simulink model "SF005A_StOutpCtrl"  (R2013b)
settings: Solver=FixedStepDiscrete  SolverMode=SingleTasking  StartTime=0.0  StopTime=1  FixedStep=0.002  RelTol=1e-3
values from neighbouring files (symbols this model uses):
  ARCHGLBPRM_2MILLISEC_SEC_F32 = DataDict.Constant    [SF005A_StOutpCtrl_DataDict.m]
  ARCHGLBPRM_FLOATZEROTHD_ULS_F32 = DataDict.Constant    [SF005A_StOutpCtrl_DataDict.m]
  BIGSLEW_ULSPERSEC_F32 = DataDict.Constant    [SF005A_StOutpCtrl_DataDict.m]
  DI_CNT_U08 = DataDict.Constant    [SF005A_StOutpCtrl_DataDict.m]
  LOA_CNT_U08 = DataDict.Constant    [SF005A_StOutpCtrl_DataDict.m]
  OPER_CNT_U08 = DataDict.Constant    [SF005A_StOutpCtrl_DataDict.m]
  STRTSTOP_CNT_U08 = DataDict.Constant    [SF005A_StOutpCtrl_DataDict.m]
libraries: NxtrLim x3, simulink x2, NxtrAbslt x1
(part 2 of 2)

== system SF005A_StOutpCtrl/StOutpCtrl/StOutpCtrlPer1/Target Selection/RateLimit ==
  note: v1.4.0: Replaced case 3 with default.
  RateSource : Inport
  OperRateLimit : Inport  Port=2
  LoaRateLimit : Inport  Port=3
  StrtStopRateLimit : Inport  Port=4
  CopyRight2 : Subsystem  Description=|  mask(Copyright Information){none=on}
      | Copyright info block.                                               
      |                                                                     
      | Place copyright information at the top of every subsystem in design.
      mask prompts: none "No parameters"
      mask help: Place copyright information at the top of every subsystem in design.
      mask Display:
      | NxtrConf = 'Nexteer Confidential';
      | 
      | sys = bdroot; %handle for the current model ("system")
      | first = get_param(sys,'Created');
      | first = first(end-3:end);  %year is last four digits
      | 
      | last = get_param(sys,'LastModifiedDate');
      | if isempty(last)
      |     last = datestr(now,'yyyy');
      | else
      |     last = last(end-3:end);
      | end
      | 
      | if strcmp(first,last)
      |     fprintf('%s -- Copyright %s Nexteer',NxtrConf,first)
      | else
      |     fprintf('%s -- %s%s- %s Nexteer',NxtrConf,char(169),first,last)
      | end
  Loa : Subsystem  TreatAsAtomicUnit=on
  Merge : Merge  Inputs=3
  Oper : Subsystem  TreatAsAtomicUnit=on
  StrtStop : Subsystem  TreatAsAtomicUnit=on
  Switch Case : SwitchCase  CaseConditions={1,2}
      settings: AttributesFormatString=|
      | Case 1: Oper
      | Case 2: Loa
      | Case 3: StrtStop
  RateLim : Outport
  wires:
  RateSource/1 -> Switch Case/1
  OperRateLimit/1 -> Oper/1(In1)
  StrtStopRateLimit/1 -> StrtStop/1(In1)
  Merge/1 -> RateLim/1  "SelectedRampRate_UlsPerSec_T_f32"
  StrtStop/1(Out1) -> Merge/1
  Loa/1(Out1) -> Merge/2
  LoaRateLimit/1 -> Loa/1(In1)
  Switch Case/1 -> Oper/Action
  Switch Case/2 -> Loa/Action
  Switch Case/3 -> StrtStop/Action
  Oper/1(Out1) -> Merge/3

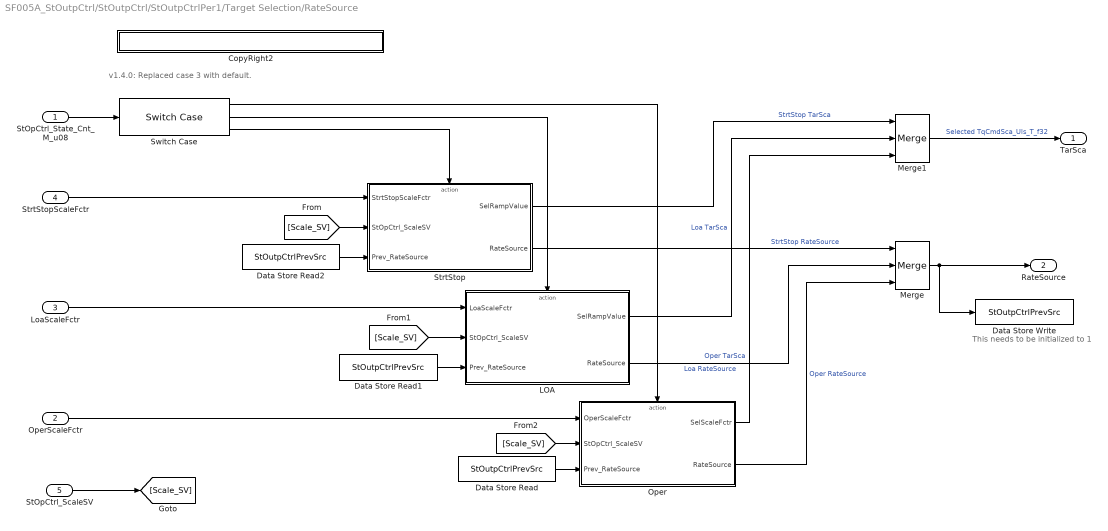
== system SF005A_StOutpCtrl/StOutpCtrl/StOutpCtrlPer1/Target Selection/RateSource ==
  note: v1.4.0: Replaced case 3 with default.
  note: This needs to be initialized to 1
  StOpCtrl_State_Cnt_M_u08 : Inport
  OperScaleFctr : Inport  Port=2
  LoaScaleFctr : Inport  Port=3
  StrtStopScaleFctr : Inport  Port=4
  StOpCtrl_ScaleSV : Inport  Port=5
  CopyRight2 : Subsystem  Description=|  mask(Copyright Information){none=on}
      | Copyright info block.                                               
      |                                                                     
      | Place copyright information at the top of every subsystem in design.
      mask prompts: none "No parameters"
      mask help: Place copyright information at the top of every subsystem in design.
      mask Display:
      | NxtrConf = 'Nexteer Confidential';
      | 
      | sys = bdroot; %handle for the current model ("system")
      | first = get_param(sys,'Created');
      | first = first(end-3:end);  %year is last four digits
      | 
      | last = get_param(sys,'LastModifiedDate');
      | if isempty(last)
      |     last = datestr(now,'yyyy');
      | else
      |     last = last(end-3:end);
      | end
      | 
      | if strcmp(first,last)
      |     fprintf('%s -- Copyright %s Nexteer',NxtrConf,first)
      | else
      |     fprintf('%s -- %s%s- %s Nexteer',NxtrConf,char(169),first,last)
      | end
  Data Store Read : DataStoreRead  DataStoreName=StOutpCtrlPrevSrc
  Data Store Read1 : DataStoreRead  DataStoreName=StOutpCtrlPrevSrc
  Data Store Read2 : DataStoreRead  DataStoreName=StOutpCtrlPrevSrc
  Data Store Write : DataStoreWrite  DataStoreName=StOutpCtrlPrevSrc
  LOA : Subsystem
  Merge : Merge  Inputs=3
  Merge1 : Merge  Inputs=3
  Oper : Subsystem
  StrtStop : Subsystem
  Switch Case : SwitchCase  CaseConditions={1,2}
      settings: AttributesFormatString=|
      | case 1: Oper
      | case 2: Loa
      | case 3: StrtStop
  TarSca : Outport
  RateSource : Outport  Port=2
  wires:
  Merge1/1 -> TarSca/1  "Selected TqCmdSca_Uls_T_f32"
  Oper/1(SelScaleFctr) -> Merge1/3  "Oper TarSca"
  LOA/2(RateSource) -> Merge/2  "Loa RateSource"
  LOA/1(SelRampValue) -> Merge1/2  "Loa TarSca"
  StrtStop/1(SelRampValue) -> Merge1/1  "StrtStop TarSca"
  Switch Case/1 -> Oper/Action
  Switch Case/2 -> LOA/Action
  Switch Case/3 -> StrtStop/Action
  Data Store Read2/1 -> StrtStop/3(Prev_RateSource)
  Data Store Read1/1 -> LOA/3(Prev_RateSource)
  [Scale_SV] -> Oper/2(StOpCtrl_ScaleSV)
  [Scale_SV] -> LOA/2(StOpCtrl_ScaleSV)
  [Scale_SV] -> StrtStop/2(StOpCtrl_ScaleSV)
  StOpCtrl_ScaleSV/1 -> [Scale_SV]
  StOpCtrl_State_Cnt_M_u08/1 -> Switch Case/1
  Oper/2(RateSource) -> Merge/3  "Oper RateSource"
  StrtStop/2(RateSource) -> Merge/1  "StrtStop RateSource"
  Merge/1 -> Data Store Write/1, RateSource/1
  StrtStopScaleFctr/1 -> StrtStop/1(StrtStopScaleFctr)
  OperScaleFctr/1 -> Oper/1(OperScaleFctr)
  LoaScaleFctr/1 -> LOA/1(LoaScaleFctr)
  Data Store Read/1 -> Oper/3(Prev_RateSource)

== system SF005A_StOutpCtrl/StOutpCtrl/StOutpCtrlPer1/Diag Override/If Action Subsystem6/CopyRight2 ==

== system SF005A_StOutpCtrl/StOutpCtrl/StOutpCtrlPer1/Diag Override/If Action Subsystem7/CopyRight2 ==

== system SF005A_StOutpCtrl/StOutpCtrl/StOutpCtrlPer1/System State Request /CtrldShtDwnFlt_FALSE/CopyRight2 ==

== system SF005A_StOutpCtrl/StOutpCtrl/StOutpCtrlPer1/System State Request /CtrldShtDwnFlt_TRUE/CopyRight2 ==

== system SF005A_StOutpCtrl/StOutpCtrl/StOutpCtrlPer1/System State Request /RampCmpl_FALSE/CopyRight2 ==

== system SF005A_StOutpCtrl/StOutpCtrl/StOutpCtrlPer1/System State Request /RampCmpl_TRUE/CopyRight2 ==

== system SF005A_StOutpCtrl/StOutpCtrl/StOutpCtrlPer1/Target Selection/RampValue/CopyRight2 ==

== system SF005A_StOutpCtrl/StOutpCtrl/StOutpCtrlPer1/Target Selection/RampValue/LOA ==
  Action Port : ActionPort  ActionType=elseif
  Constant1 : Constant  Value=LOA_CNT_U08  OutDataTypeStr=uint8
      settings: AttributesFormatString=%<OutDataTypeStr>
  CopyRight2 : Subsystem  Description=|  mask(Copyright Information){none=on}
      | Copyright info block.                                               
      |                                                                     
      | Place copyright information at the top of every subsystem in design.
      mask prompts: none "No parameters"
      mask help: Place copyright information at the top of every subsystem in design.
      mask Display:
      | NxtrConf = 'Nexteer Confidential';
      | 
      | sys = bdroot; %handle for the current model ("system")
      | first = get_param(sys,'Created');
      | first = first(end-3:end);  %year is last four digits
      | 
      | last = get_param(sys,'LastModifiedDate');
      | if isempty(last)
      |     last = datestr(now,'yyyy');
      | else
      |     last = last(end-3:end);
      | end
      | 
      | if strcmp(first,last)
      |     fprintf('%s -- Copyright %s Nexteer',NxtrConf,first)
      | else
      |     fprintf('%s -- %s%s- %s Nexteer',NxtrConf,char(169),first,last)
      | end
  Out1 : Outport
  wires:
  Constant1/1 -> Out1/1

== system SF005A_StOutpCtrl/StOutpCtrl/StOutpCtrlPer1/Target Selection/RampValue/Oper ==
  Action Port : ActionPort  ActionType=else
  Constant : Constant  Value=OPER_CNT_U08  OutDataTypeStr=uint8
      settings: AttributesFormatString=%<OutDataTypeStr>
  CopyRight2 : Subsystem  Description=|  mask(Copyright Information){none=on}
      | Copyright info block.                                               
      |                                                                     
      | Place copyright information at the top of every subsystem in design.
      mask prompts: none "No parameters"
      mask help: Place copyright information at the top of every subsystem in design.
      mask Display:
      | NxtrConf = 'Nexteer Confidential';
      | 
      | sys = bdroot; %handle for the current model ("system")
      | first = get_param(sys,'Created');
      | first = first(end-3:end);  %year is last four digits
      | 
      | last = get_param(sys,'LastModifiedDate');
      | if isempty(last)
      |     last = datestr(now,'yyyy');
      | else
      |     last = last(end-3:end);
      | end
      | 
      | if strcmp(first,last)
      |     fprintf('%s -- Copyright %s Nexteer',NxtrConf,first)
      | else
      |     fprintf('%s -- %s%s- %s Nexteer',NxtrConf,char(169),first,last)
      | end
  Out1 : Outport
  wires:
  Constant/1 -> Out1/1

== system SF005A_StOutpCtrl/StOutpCtrl/StOutpCtrlPer1/Target Selection/RampValue/StrtStop ==
  Action Port : ActionPort  ActionType=then
  Constant2 : Constant  Value=STRTSTOP_CNT_U08  OutDataTypeStr=uint8
      settings: AttributesFormatString=%<OutDataTypeStr>
  CopyRight2 : Subsystem  Description=|  mask(Copyright Information){none=on}
      | Copyright info block.                                               
      |                                                                     
      | Place copyright information at the top of every subsystem in design.
      mask prompts: none "No parameters"
      mask help: Place copyright information at the top of every subsystem in design.
      mask Display:
      | NxtrConf = 'Nexteer Confidential';
      | 
      | sys = bdroot; %handle for the current model ("system")
      | first = get_param(sys,'Created');
      | first = first(end-3:end);  %year is last four digits
      | 
      | last = get_param(sys,'LastModifiedDate');
      | if isempty(last)
      |     last = datestr(now,'yyyy');
      | else
      |     last = last(end-3:end);
      | end
      | 
      | if strcmp(first,last)
      |     fprintf('%s -- Copyright %s Nexteer',NxtrConf,first)
      | else
      |     fprintf('%s -- %s%s- %s Nexteer',NxtrConf,char(169),first,last)
      | end
  Out1 : Outport
  wires:
  Constant2/1 -> Out1/1

== system SF005A_StOutpCtrl/StOutpCtrl/StOutpCtrlPer1/Target Selection/RateLimit/CopyRight2 ==

== system SF005A_StOutpCtrl/StOutpCtrl/StOutpCtrlPer1/Target Selection/RateLimit/Loa ==
  In1 : Inport
  Action Port : ActionPort  ActionType=case
  CopyRight2 : Subsystem  Description=|  mask(Copyright Information){none=on}
      | Copyright info block.                                               
      |                                                                     
      | Place copyright information at the top of every subsystem in design.
      mask prompts: none "No parameters"
      mask help: Place copyright information at the top of every subsystem in design.
      mask Display:
      | NxtrConf = 'Nexteer Confidential';
      | 
      | sys = bdroot; %handle for the current model ("system")
      | first = get_param(sys,'Created');
      | first = first(end-3:end);  %year is last four digits
      | 
      | last = get_param(sys,'LastModifiedDate');
      | if isempty(last)
      |     last = datestr(now,'yyyy');
      | else
      |     last = last(end-3:end);
      | end
      | 
      | if strcmp(first,last)
      |     fprintf('%s -- Copyright %s Nexteer',NxtrConf,first)
      | else
      |     fprintf('%s -- %s%s- %s Nexteer',NxtrConf,char(169),first,last)
      | end
  Out1 : Outport
  wires:
  In1/1 -> Out1/1

== system SF005A_StOutpCtrl/StOutpCtrl/StOutpCtrlPer1/Target Selection/RateLimit/Oper ==
  In1 : Inport
  Action Port : ActionPort  ActionType=case
  CopyRight2 : Subsystem  Description=|  mask(Copyright Information){none=on}
      | Copyright info block.                                               
      |                                                                     
      | Place copyright information at the top of every subsystem in design.
      mask prompts: none "No parameters"
      mask help: Place copyright information at the top of every subsystem in design.
      mask Display:
      | NxtrConf = 'Nexteer Confidential';
      | 
      | sys = bdroot; %handle for the current model ("system")
      | first = get_param(sys,'Created');
      | first = first(end-3:end);  %year is last four digits
      | 
      | last = get_param(sys,'LastModifiedDate');
      | if isempty(last)
      |     last = datestr(now,'yyyy');
      | else
      |     last = last(end-3:end);
      | end
      | 
      | if strcmp(first,last)
      |     fprintf('%s -- Copyright %s Nexteer',NxtrConf,first)
      | else
      |     fprintf('%s -- %s%s- %s Nexteer',NxtrConf,char(169),first,last)
      | end
  Out1 : Outport
  wires:
  In1/1 -> Out1/1

== system SF005A_StOutpCtrl/StOutpCtrl/StOutpCtrlPer1/Target Selection/RateLimit/StrtStop ==
  In1 : Inport
  Action Port : ActionPort  ActionType=case
  CopyRight2 : Subsystem  Description=|  mask(Copyright Information){none=on}
      | Copyright info block.                                               
      |                                                                     
      | Place copyright information at the top of every subsystem in design.
      mask prompts: none "No parameters"
      mask help: Place copyright information at the top of every subsystem in design.
      mask Display:
      | NxtrConf = 'Nexteer Confidential';
      | 
      | sys = bdroot; %handle for the current model ("system")
      | first = get_param(sys,'Created');
      | first = first(end-3:end);  %year is last four digits
      | 
      | last = get_param(sys,'LastModifiedDate');
      | if isempty(last)
      |     last = datestr(now,'yyyy');
      | else
      |     last = last(end-3:end);
      | end
      | 
      | if strcmp(first,last)
      |     fprintf('%s -- Copyright %s Nexteer',NxtrConf,first)
      | else
      |     fprintf('%s -- %s%s- %s Nexteer',NxtrConf,char(169),first,last)
      | end
  Out1 : Outport
  wires:
  In1/1 -> Out1/1

== system SF005A_StOutpCtrl/StOutpCtrl/StOutpCtrlPer1/Target Selection/RateSource/CopyRight2 ==

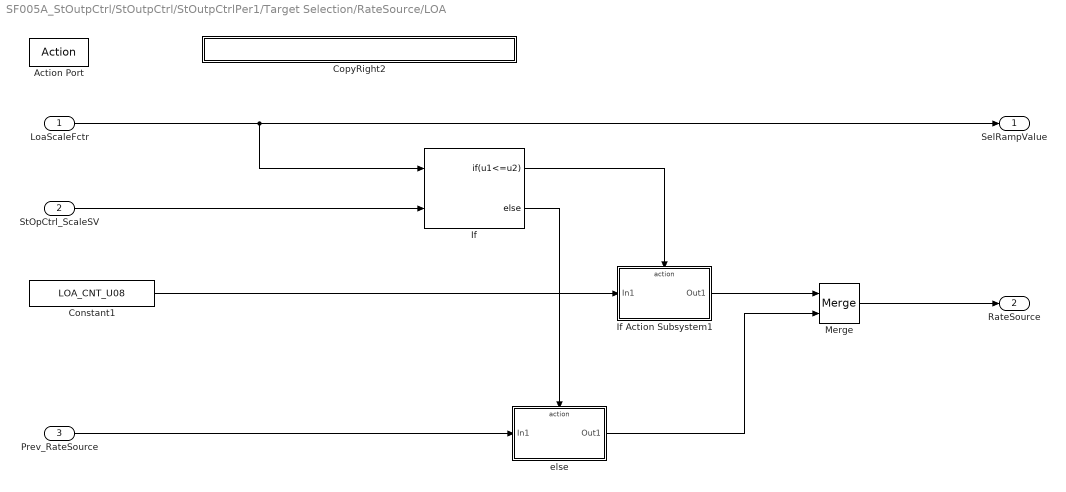
== system SF005A_StOutpCtrl/StOutpCtrl/StOutpCtrlPer1/Target Selection/RateSource/LOA ==
  LoaScaleFctr : Inport
  StOpCtrl_ScaleSV : Inport  Port=2
  Prev_RateSource : Inport  Port=3
  Action Port : ActionPort  ActionType=case
  Constant1 : Constant  Value=LOA_CNT_U08  OutDataTypeStr=uint8
      settings: AttributesFormatString=%<OutDataTypeStr>
  CopyRight2 : Subsystem  Description=|  mask(Copyright Information){none=on}
      | Copyright info block.                                               
      |                                                                     
      | Place copyright information at the top of every subsystem in design.
      mask prompts: none "No parameters"
      mask help: Place copyright information at the top of every subsystem in design.
      mask Display:
      | NxtrConf = 'Nexteer Confidential';
      | 
      | sys = bdroot; %handle for the current model ("system")
      | first = get_param(sys,'Created');
      | first = first(end-3:end);  %year is last four digits
      | 
      | last = get_param(sys,'LastModifiedDate');
      | if isempty(last)
      |     last = datestr(now,'yyyy');
      | else
      |     last = last(end-3:end);
      | end
      | 
      | if strcmp(first,last)
      |     fprintf('%s -- Copyright %s Nexteer',NxtrConf,first)
      | else
      |     fprintf('%s -- %s%s- %s Nexteer',NxtrConf,char(169),first,last)
      | end
  If : If  RequirementInfo={'linktype_rmi_doors' '0000baae (/E-STEER Core/SubSystem Specifications/Application Functions/SF005A State Output Control)' '#SF005A_54' 'true' 'REQ: SF005A_54' '' ; 'linktype_rmi_doors' '0000baae (/E-STEER Core/SubSystem Specifications/Application Functions/SF005A State Output Control)' '#SF005A_55' 'true' 'REQ: SF005A_55' '' ; 'linktype_rmi_doors' '0000baae (/E-STEER Core/SubSystem Specifications/Application Functions/SF005A State Output Control)' '#SF005A_61' 'true' 'REQ: SF005A_61' '' } %GIDa_5c692240_752d_457b_a676_1ce9a35b4c5b  NumInputs=2  IfExpression=u1<=u2
  If Action Subsystem1 : Subsystem  TreatAsAtomicUnit=on
  Merge : Merge
  else : Subsystem  TreatAsAtomicUnit=on
  SelRampValue : Outport
  RateSource : Outport  Port=2
  wires:
  If Action Subsystem1/1(Out1) -> Merge/1
  else/1(Out1) -> Merge/2
  Merge/1 -> RateSource/1
  Prev_RateSource/1 -> else/1(In1)
  If/2 -> else/Action
  Constant1/1 -> If Action Subsystem1/1(In1)
  StOpCtrl_ScaleSV/1 -> If/2
  If/1 -> If Action Subsystem1/Action
  LoaScaleFctr/1 -> If/1, SelRampValue/1

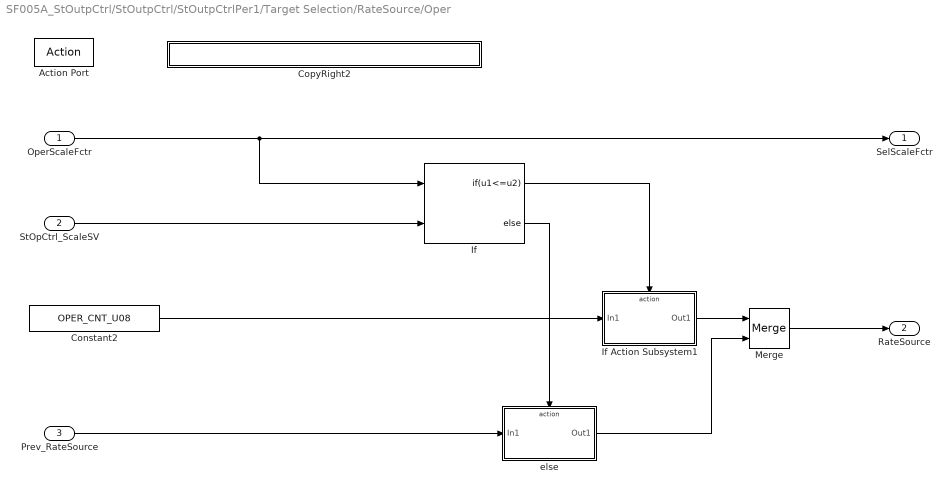
== system SF005A_StOutpCtrl/StOutpCtrl/StOutpCtrlPer1/Target Selection/RateSource/Oper ==
  OperScaleFctr : Inport
  StOpCtrl_ScaleSV : Inport  Port=2
  Prev_RateSource : Inport  Port=3
  Action Port : ActionPort  ActionType=case
  Constant2 : Constant  Value=OPER_CNT_U08  OutDataTypeStr=uint8
      settings: AttributesFormatString=%<OutDataTypeStr>
  CopyRight2 : Subsystem  Description=|  mask(Copyright Information){none=on}
      | Copyright info block.                                               
      |                                                                     
      | Place copyright information at the top of every subsystem in design.
      mask prompts: none "No parameters"
      mask help: Place copyright information at the top of every subsystem in design.
      mask Display:
      | NxtrConf = 'Nexteer Confidential';
      | 
      | sys = bdroot; %handle for the current model ("system")
      | first = get_param(sys,'Created');
      | first = first(end-3:end);  %year is last four digits
      | 
      | last = get_param(sys,'LastModifiedDate');
      | if isempty(last)
      |     last = datestr(now,'yyyy');
      | else
      |     last = last(end-3:end);
      | end
      | 
      | if strcmp(first,last)
      |     fprintf('%s -- Copyright %s Nexteer',NxtrConf,first)
      | else
      |     fprintf('%s -- %s%s- %s Nexteer',NxtrConf,char(169),first,last)
      | end
  If : If  RequirementInfo={'linktype_rmi_doors' '0000baae (/E-STEER Core/SubSystem Specifications/Application Functions/SF005A State Output Control)' '#SF005A_54' 'true' 'REQ: SF005A_54' '' ; 'linktype_rmi_doors' '0000baae (/E-STEER Core/SubSystem Specifications/Application Functions/SF005A State Output Control)' '#SF005A_55' 'true' 'REQ: SF005A_55' '' ; 'linktype_rmi_doors' '0000baae (/E-STEER Core/SubSystem Specifications/Application Functions/SF005A State Output Control)' '#SF005A_61' 'true' 'REQ: SF005A_61' '' } %GIDa_7f0fcea9_e623_490b_b477_8070bf8ccca9  NumInputs=2  IfExpression=u1<=u2
  If Action Subsystem1 : Subsystem  TreatAsAtomicUnit=on
  Merge : Merge
  else : Subsystem  TreatAsAtomicUnit=on
  SelScaleFctr : Outport
  RateSource : Outport  Port=2
  wires:
  else/1(Out1) -> Merge/2
  If Action Subsystem1/1(Out1) -> Merge/1
  Merge/1 -> RateSource/1
  Prev_RateSource/1 -> else/1(In1)
  If/2 -> else/Action
  Constant2/1 -> If Action Subsystem1/1(In1)
  StOpCtrl_ScaleSV/1 -> If/2
  If/1 -> If Action Subsystem1/Action
  OperScaleFctr/1 -> If/1, SelScaleFctr/1

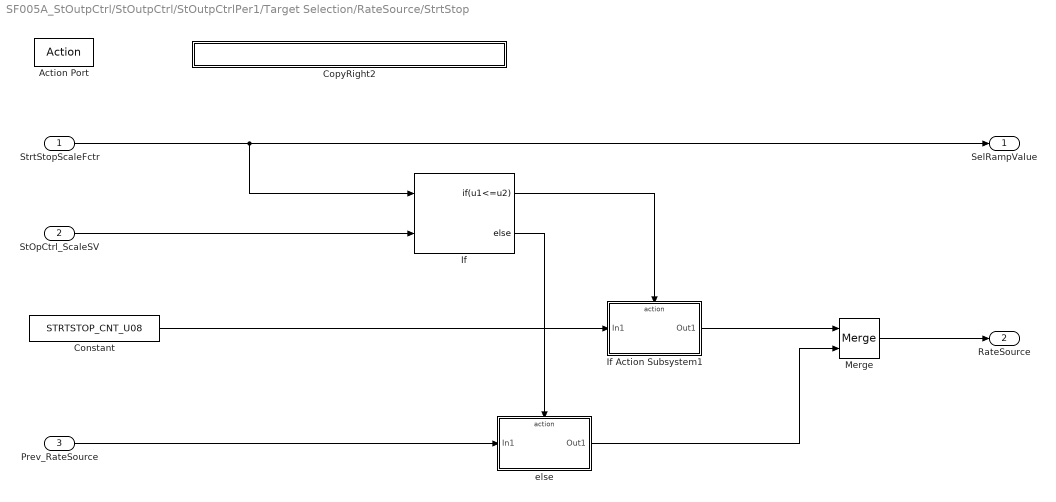
== system SF005A_StOutpCtrl/StOutpCtrl/StOutpCtrlPer1/Target Selection/RateSource/StrtStop ==
  StrtStopScaleFctr : Inport
  StOpCtrl_ScaleSV : Inport  Port=2
  Prev_RateSource : Inport  Port=3
  Action Port : ActionPort  ActionType=case
  Constant : Constant  Value=STRTSTOP_CNT_U08  OutDataTypeStr=uint8
      settings: AttributesFormatString=%<OutDataTypeStr>
  CopyRight2 : Subsystem  Description=|  mask(Copyright Information){none=on}
      | Copyright info block.                                               
      |                                                                     
      | Place copyright information at the top of every subsystem in design.
      mask prompts: none "No parameters"
      mask help: Place copyright information at the top of every subsystem in design.
      mask Display:
      | NxtrConf = 'Nexteer Confidential';
      | 
      | sys = bdroot; %handle for the current model ("system")
      | first = get_param(sys,'Created');
      | first = first(end-3:end);  %year is last four digits
      | 
      | last = get_param(sys,'LastModifiedDate');
      | if isempty(last)
      |     last = datestr(now,'yyyy');
      | else
      |     last = last(end-3:end);
      | end
      | 
      | if strcmp(first,last)
      |     fprintf('%s -- Copyright %s Nexteer',NxtrConf,first)
      | else
      |     fprintf('%s -- %s%s- %s Nexteer',NxtrConf,char(169),first,last)
      | end
  If : If  RequirementInfo={'linktype_rmi_doors' '0000baae (/E-STEER Core/SubSystem Specifications/Application Functions/SF005A State Output Control)' '#SF005A_54' 'true' 'REQ: SF005A_54' '' ; 'linktype_rmi_doors' '0000baae (/E-STEER Core/SubSystem Specifications/Application Functions/SF005A State Output Control)' '#SF005A_55' 'true' 'REQ: SF005A_55' '' ; 'linktype_rmi_doors' '0000baae (/E-STEER Core/SubSystem Specifications/Application Functions/SF005A State Output Control)' '#SF005A_61' 'true' 'REQ: SF005A_61' '' } %GIDa_2d9fc241_76de_4798_baaf_ed414e6e2a48  NumInputs=2  IfExpression=u1<=u2
  If Action Subsystem1 : Subsystem  TreatAsAtomicUnit=on
  Merge : Merge
  else : Subsystem  TreatAsAtomicUnit=on
  SelRampValue : Outport
  RateSource : Outport  Port=2
  wires:
  else/1(Out1) -> Merge/2
  If Action Subsystem1/1(Out1) -> Merge/1
  Merge/1 -> RateSource/1
  Prev_RateSource/1 -> else/1(In1)
  If/2 -> else/Action
  StOpCtrl_ScaleSV/1 -> If/2
  If/1 -> If Action Subsystem1/Action
  StrtStopScaleFctr/1 -> If/1, SelRampValue/1
  Constant/1 -> If Action Subsystem1/1(In1)

== system SF005A_StOutpCtrl/StOutpCtrl/StOutpCtrlPer1/Target Selection/RampValue/LOA/CopyRight2 ==

== system SF005A_StOutpCtrl/StOutpCtrl/StOutpCtrlPer1/Target Selection/RampValue/Oper/CopyRight2 ==

== system SF005A_StOutpCtrl/StOutpCtrl/StOutpCtrlPer1/Target Selection/RampValue/StrtStop/CopyRight2 ==

== system SF005A_StOutpCtrl/StOutpCtrl/StOutpCtrlPer1/Target Selection/RateLimit/Loa/CopyRight2 ==

== system SF005A_StOutpCtrl/StOutpCtrl/StOutpCtrlPer1/Target Selection/RateLimit/Oper/CopyRight2 ==

== system SF005A_StOutpCtrl/StOutpCtrl/StOutpCtrlPer1/Target Selection/RateLimit/StrtStop/CopyRight2 ==

== system SF005A_StOutpCtrl/StOutpCtrl/StOutpCtrlPer1/Target Selection/RateSource/LOA/CopyRight2 ==

== system SF005A_StOutpCtrl/StOutpCtrl/StOutpCtrlPer1/Target Selection/RateSource/LOA/If Action Subsystem1 ==
  In1 : Inport
  Action Port : ActionPort  ActionType=then
  CopyRight2 : Subsystem  Description=|  mask(Copyright Information){none=on}
      | Copyright info block.                                               
      |                                                                     
      | Place copyright information at the top of every subsystem in design.
      mask prompts: none "No parameters"
      mask help: Place copyright information at the top of every subsystem in design.
      mask Display:
      | NxtrConf = 'Nexteer Confidential';
      | 
      | sys = bdroot; %handle for the current model ("system")
      | first = get_param(sys,'Created');
      | first = first(end-3:end);  %year is last four digits
      | 
      | last = get_param(sys,'LastModifiedDate');
      | if isempty(last)
      |     last = datestr(now,'yyyy');
      | else
      |     last = last(end-3:end);
      | end
      | 
      | if strcmp(first,last)
      |     fprintf('%s -- Copyright %s Nexteer',NxtrConf,first)
      | else
      |     fprintf('%s -- %s%s- %s Nexteer',NxtrConf,char(169),first,last)
      | end
  Out1 : Outport
  wires:
  In1/1 -> Out1/1

== system SF005A_StOutpCtrl/StOutpCtrl/StOutpCtrlPer1/Target Selection/RateSource/LOA/else ==
  In1 : Inport
  Action Port : ActionPort  ActionType=else
  CopyRight2 : Subsystem  Description=|  mask(Copyright Information){none=on}
      | Copyright info block.                                               
      |                                                                     
      | Place copyright information at the top of every subsystem in design.
      mask prompts: none "No parameters"
      mask help: Place copyright information at the top of every subsystem in design.
      mask Display:
      | NxtrConf = 'Nexteer Confidential';
      | 
      | sys = bdroot; %handle for the current model ("system")
      | first = get_param(sys,'Created');
      | first = first(end-3:end);  %year is last four digits
      | 
      | last = get_param(sys,'LastModifiedDate');
      | if isempty(last)
      |     last = datestr(now,'yyyy');
      | else
      |     last = last(end-3:end);
      | end
      | 
      | if strcmp(first,last)
      |     fprintf('%s -- Copyright %s Nexteer',NxtrConf,first)
      | else
      |     fprintf('%s -- %s%s- %s Nexteer',NxtrConf,char(169),first,last)
      | end
  Out1 : Outport
  wires:
  In1/1 -> Out1/1

== system SF005A_StOutpCtrl/StOutpCtrl/StOutpCtrlPer1/Target Selection/RateSource/Oper/CopyRight2 ==

== system SF005A_StOutpCtrl/StOutpCtrl/StOutpCtrlPer1/Target Selection/RateSource/Oper/If Action Subsystem1 ==
  In1 : Inport
  Action Port : ActionPort  ActionType=then
  CopyRight2 : Subsystem  Description=|  mask(Copyright Information){none=on}
      | Copyright info block.                                               
      |                                                                     
      | Place copyright information at the top of every subsystem in design.
      mask prompts: none "No parameters"
      mask help: Place copyright information at the top of every subsystem in design.
      mask Display:
      | NxtrConf = 'Nexteer Confidential';
      | 
      | sys = bdroot; %handle for the current model ("system")
      | first = get_param(sys,'Created');
      | first = first(end-3:end);  %year is last four digits
      | 
      | last = get_param(sys,'LastModifiedDate');
      | if isempty(last)
      |     last = datestr(now,'yyyy');
      | else
      |     last = last(end-3:end);
      | end
      | 
      | if strcmp(first,last)
      |     fprintf('%s -- Copyright %s Nexteer',NxtrConf,first)
      | else
      |     fprintf('%s -- %s%s- %s Nexteer',NxtrConf,char(169),first,last)
      | end
  Out1 : Outport
  wires:
  In1/1 -> Out1/1

== system SF005A_StOutpCtrl/StOutpCtrl/StOutpCtrlPer1/Target Selection/RateSource/Oper/else ==
  In1 : Inport
  Action Port : ActionPort  ActionType=else
  CopyRight2 : Subsystem  Description=|  mask(Copyright Information){none=on}
      | Copyright info block.                                               
      |                                                                     
      | Place copyright information at the top of every subsystem in design.
      mask prompts: none "No parameters"
      mask help: Place copyright information at the top of every subsystem in design.
      mask Display:
      | NxtrConf = 'Nexteer Confidential';
      | 
      | sys = bdroot; %handle for the current model ("system")
      | first = get_param(sys,'Created');
      | first = first(end-3:end);  %year is last four digits
      | 
      | last = get_param(sys,'LastModifiedDate');
      | if isempty(last)
      |     last = datestr(now,'yyyy');
      | else
      |     last = last(end-3:end);
      | end
      | 
      | if strcmp(first,last)
      |     fprintf('%s -- Copyright %s Nexteer',NxtrConf,first)
      | else
      |     fprintf('%s -- %s%s- %s Nexteer',NxtrConf,char(169),first,last)
      | end
  Out1 : Outport
  wires:
  In1/1 -> Out1/1

== system SF005A_StOutpCtrl/StOutpCtrl/StOutpCtrlPer1/Target Selection/RateSource/StrtStop/CopyRight2 ==

== system SF005A_StOutpCtrl/StOutpCtrl/StOutpCtrlPer1/Target Selection/RateSource/StrtStop/If Action Subsystem1 ==
  In1 : Inport
  Action Port : ActionPort  ActionType=then
  CopyRight2 : Subsystem  Description=|  mask(Copyright Information){none=on}
      | Copyright info block.                                               
      |                                                                     
      | Place copyright information at the top of every subsystem in design.
      mask prompts: none "No parameters"
      mask help: Place copyright information at the top of every subsystem in design.
      mask Display:
      | NxtrConf = 'Nexteer Confidential';
      | 
      | sys = bdroot; %handle for the current model ("system")
      | first = get_param(sys,'Created');
      | first = first(end-3:end);  %year is last four digits
      | 
      | last = get_param(sys,'LastModifiedDate');
      | if isempty(last)
      |     last = datestr(now,'yyyy');
      | else
      |     last = last(end-3:end);
      | end
      | 
      | if strcmp(first,last)
      |     fprintf('%s -- Copyright %s Nexteer',NxtrConf,first)
      | else
      |     fprintf('%s -- %s%s- %s Nexteer',NxtrConf,char(169),first,last)
      | end
  Out1 : Outport
  wires:
  In1/1 -> Out1/1

== system SF005A_StOutpCtrl/StOutpCtrl/StOutpCtrlPer1/Target Selection/RateSource/StrtStop/else ==
  In1 : Inport
  Action Port : ActionPort  ActionType=else
  CopyRight2 : Subsystem  Description=|  mask(Copyright Information){none=on}
      | Copyright info block.                                               
      |                                                                     
      | Place copyright information at the top of every subsystem in design.
      mask prompts: none "No parameters"
      mask help: Place copyright information at the top of every subsystem in design.
      mask Display:
      | NxtrConf = 'Nexteer Confidential';
      | 
      | sys = bdroot; %handle for the current model ("system")
      | first = get_param(sys,'Created');
      | first = first(end-3:end);  %year is last four digits
      | 
      | last = get_param(sys,'LastModifiedDate');
      | if isempty(last)
      |     last = datestr(now,'yyyy');
      | else
      |     last = last(end-3:end);
      | end
      | 
      | if strcmp(first,last)
      |     fprintf('%s -- Copyright %s Nexteer',NxtrConf,first)
      | else
      |     fprintf('%s -- %s%s- %s Nexteer',NxtrConf,char(169),first,last)
      | end
  Out1 : Outport
  wires:
  In1/1 -> Out1/1

== system SF005A_StOutpCtrl/StOutpCtrl/StOutpCtrlPer1/Target Selection/RateSource/LOA/If Action Subsystem1/CopyRight2 ==

== system SF005A_StOutpCtrl/StOutpCtrl/StOutpCtrlPer1/Target Selection/RateSource/LOA/else/CopyRight2 ==

== system SF005A_StOutpCtrl/StOutpCtrl/StOutpCtrlPer1/Target Selection/RateSource/Oper/If Action Subsystem1/CopyRight2 ==

== system SF005A_StOutpCtrl/StOutpCtrl/StOutpCtrlPer1/Target Selection/RateSource/Oper/else/CopyRight2 ==

== system SF005A_StOutpCtrl/StOutpCtrl/StOutpCtrlPer1/Target Selection/RateSource/StrtStop/If Action Subsystem1/CopyRight2 ==

== system SF005A_StOutpCtrl/StOutpCtrl/StOutpCtrlPer1/Target Selection/RateSource/StrtStop/else/CopyRight2 ==
